simulink model "PLL_Lock_sim"  (R2021b)
settings: Solver=ode23tb  StartTime=0.0  StopTime=3.000e+00  RelTol=1e-3
model workspace (MAT data in the model file):
  Frequency_12 = 99994730.511
  LockTime_12 = 0
  PhaseNoise_12 = [-24.1905770852 -116.991131031 -135.719436806 -153.68193214 -165.966096628]
  PnFrequencyOffset_12 = [2 300000 1000000 3000000 10000000]
  TargetFrequency_12 = 100000000
  TargetLockTime_12 = 3e-06
  TargetPhaseNoise_12 = [-70 -85 -125 -150 -180]
  uniqueStringPll_12 = '97_0593'
  uniqueString_12 = '95_7167'
libraries: msbPllFoundation x5, msbPllMeasurements x1
settings Model: SimulationMode=accelerator  Creator=Eins  LastModifiedBy=Eins

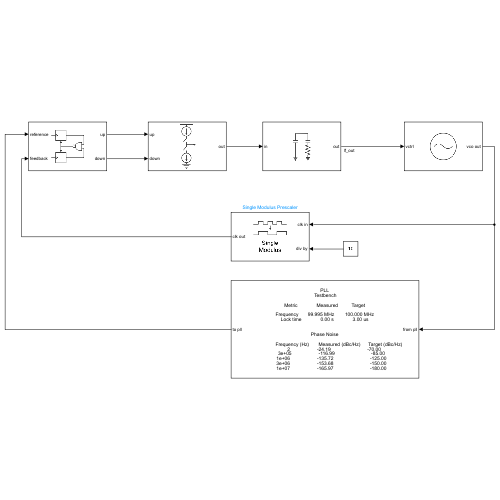
[thumbnail: Simulink's stored preview of the top-level diagram]
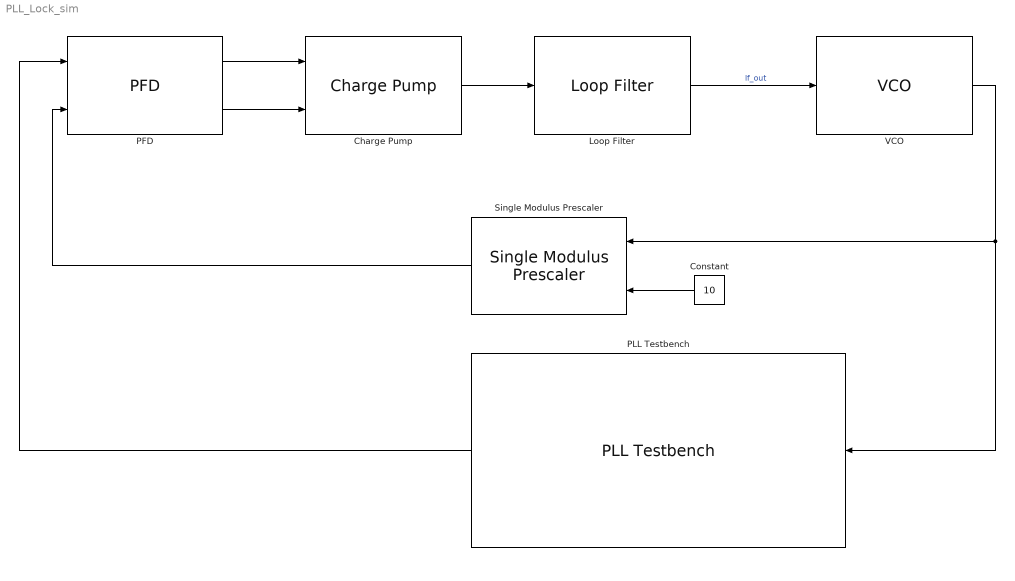
== system PLL_Lock_sim ==
  Charge Pump : msbPllFoundation/Charge Pump  OutputCurrent=5e-3  InputThreshold=0.5  ExtraBuffer=off  NBuffer=10  EnableCurrentImpairments=on  CurrentImbalance=1e-7  LeakageCurrent=1e-8  EnableTimingImpairments=on  DefaultOrAdvanced=Default  MaxFreqInterest=10e9  RiseFallUp=5e-9  PropDelayUp=6e-9  RiseFallDown=2e-9  PropDelayDown=4e-9
      settings: SourceProductBaseCode=AM
  Constant : Constant  Value=10
  Loop Filter : msbPllFoundation/Loop Filter  FilterType=2nd order passive  C1=82e-9  C2=1e-6  C3=1.0452e-15  C4=1e-12  R2=56e3  R3=51.0435e6  R4=12e3  ExtraBuffer=off  NBuffer=1000  EnableImpairments=off  Temperature=30
      settings: SourceProductBaseCode=AM
  PFD : msbPllFoundation/PFD  DeadbandCompensation=30e-12  ExtraBuffer=off  NBuffer=10  EnableImpairments=on  DefaultOrAdvanced=Default  MaxFreqInterest=10e9  RiseFallTime=30e-12  PropDelay=50e-12
      settings: SourceProductBaseCode=AM
  PLL Testbench : msbPllMeasurements/PLL Testbench  InputAmplitude=1  ClkFreq=10e6  FrequencyMeasureOption=on  CurrentFrequency=0  LockTimeOption=on  ExpectedFreq=100e6  FreqErrorTol=100  CurrentLockTime=0  PhaseNoiseOption=on  SampleRate=8*2e9  ResBandwidth=2  SpectralAverages=4  HoldOffTime=0  PhaseNoiseFreqOffset=[2 300e3 1e6 3e6 10e6]  OpenSpectrum=off  ExtraBuffer=off  NBuffer=0  PowerVector=0  FrequencyVector=0  TargetFreq=2.1e9  TargetLockTime=3e-6  TargetPhaseNoiseVector=[-70,-85,-125,-150,-180]
      settings: SourceProductBaseCode=AM  SignalType=Square
  Single Modulus Prescaler : msbPllFoundation/Single Modulus Prescaler  ExtraBuffer=off  NBuffer=1
      settings: SourceProductBaseCode=AM
  VCO : msbPllFoundation/VCO  SpecifyUsing=Voltage sensitivity  Kvco=2  Fo=99.999995e6  ControlVoltage=[-5 0 5]  OutputFrequency=[2e9 2.5e9 3e9]  Amplitude=0.4  ExtraBuffer=off  NBuffer=10  AddPhaseNoise=on  Foffset=[30e3 100e3 1e6 3e6 10e6]  PhaseNoise=[-56 -106 -132 -143 -152]  MaxKvco=2
      settings: SourceProductBaseCode=AM
  wires:
  PFD/1 -> Charge Pump/1
  PFD/2 -> Charge Pump/2
  Charge Pump/1 -> Loop Filter/1
  Loop Filter/1 -> VCO/1  "lf_out"
  VCO/1 -> PLL Testbench/1, Single Modulus Prescaler/1
  Single Modulus Prescaler/1 -> PFD/2
  Constant/1 -> Single Modulus Prescaler/2
  PLL Testbench/1 -> PFD/1
